simulink model "Intergration"  (R2018b)
settings: Solver=FixedStepDiscrete  StartTime=0.0  StopTime=inf  FixedStep=0.005  RelTol=1e-3
PostLoadFcn:
  | if any(exist('dsrtsu_mdlpostloadfcn', 'file') ~= 0), dsrtsu_mdlpostloadfcn('Execute', bdroot); end
values from neighbouring files (symbols this model uses):
  P_x165_On = 1.0    [CAN_Tx.sldd]
  P_x242_On = 1.0    [CAN_Tx.sldd]
  P_x246_On = 1.0    [CAN_Tx.sldd]
libraries: rtican x112, simulink x59
(part 29 of 31)

== system Intergration/Radar410_RX/Subsystem41/Subsystem29 ==
  In1 : Inport
  Bus Creator : BusCreator  Inputs=20  OutDataTypeStr=Bus: Obj_Data  NonVirtualBus=on
      settings: InheritFromInputs=off
  Bus Selector : BusSelector  OutputSignals=FRS_P1_27_Msg_CheckSum,FRS_P1_27_Msg_AliveCounter,FRS_P1_27_Obj_ExstProb,FRS_P1_27_Obj_XVelRel_Stdev,FRS_P1_27_Obj_XAccRel,FRS_P1_27_Obj_ObstacleProb,FRS_P1_27_Obj_MotionPattern,FRS_P1_27_Obj_YPos_Stdev,FRS_P1_27_Obj_ValidFlag,FRS_P1_27_Obj_XPos_Stdev,FRS_P1_27_Obj_UpdateFlag,FRS_P1_27_Obj_ID,FRS_P2_27_Msg_CheckSum,FRS_P2_27_Msg_AliveCounter,FRS_P2_27_Obj_MeasFlag,FRS_P2_27_Obj_YVelRel,FRS_P2_27_Obj_Type,FRS_P2_27_Obj_XPos,FRS_P2_27_Obj_YPos,FRS_P2_27_Obj_XVelRel
  Data Type Conversion{,1..19} (20 alike) : DataTypeConversion  OutDataTypeStr=single
  Out1 : Outport  OutDataTypeStr=Bus: Obj_Data
  wires:
  Data Type Conversion12/1 -> Bus Creator/13
  Bus Selector/5 -> Data Type Conversion4/1  "<FRS_P1_27_Obj_XAccRel>"
  Bus Selector/8 -> Data Type Conversion7/1  "<FRS_P1_27_Obj_YPos_Stdev>"
  Data Type Conversion15/1 -> Bus Creator/16
  Bus Selector/1 -> Data Type Conversion/1  "<FRS_P1_27_Msg_CheckSum>"
  Bus Selector/15 -> Data Type Conversion14/1  "<FRS_P2_27_Obj_MeasFlag>"
  Bus Selector/3 -> Data Type Conversion2/1  "<FRS_P1_27_Obj_ExstProb>"
  Bus Selector/13 -> Data Type Conversion12/1  "<FRS_P2_27_Msg_CheckSum>"
  Bus Selector/2 -> Data Type Conversion1/1  "<FRS_P1_27_Msg_AliveCounter>"
  Data Type Conversion11/1 -> Bus Creator/12
  Data Type Conversion5/1 -> Bus Creator/6
  Bus Selector/4 -> Data Type Conversion3/1  "<FRS_P1_27_Obj_XVelRel_Stdev>"
  Bus Selector/7 -> Data Type Conversion6/1  "<FRS_P1_27_Obj_MotionPattern>"
  Data Type Conversion9/1 -> Bus Creator/10
  Bus Selector/6 -> Data Type Conversion5/1  "<FRS_P1_27_Obj_ObstacleProb>"
  Data Type Conversion18/1 -> Bus Creator/19
  Bus Selector/11 -> Data Type Conversion10/1  "<FRS_P1_27_Obj_UpdateFlag>"
  Data Type Conversion17/1 -> Bus Creator/18
  Bus Selector/16 -> Data Type Conversion15/1  "<FRS_P2_27_Obj_YVelRel>"
  Data Type Conversion6/1 -> Bus Creator/7
  Bus Selector/12 -> Data Type Conversion11/1  "<FRS_P1_27_Obj_ID>"
  Data Type Conversion16/1 -> Bus Creator/17
  Bus Selector/9 -> Data Type Conversion8/1  "<FRS_P1_27_Obj_ValidFlag>"
  Bus Selector/17 -> Data Type Conversion16/1  "<FRS_P2_27_Obj_Type>"
  Bus Selector/10 -> Data Type Conversion9/1  "<FRS_P1_27_Obj_XPos_Stdev>"
  Data Type Conversion10/1 -> Bus Creator/11
  Bus Selector/14 -> Data Type Conversion13/1  "<FRS_P2_27_Msg_AliveCounter>"
  Bus Selector/19 -> Data Type Conversion18/1  "<FRS_P2_27_Obj_YPos>"
  Bus Selector/18 -> Data Type Conversion17/1  "<FRS_P2_27_Obj_XPos>"
  Bus Selector/20 -> Data Type Conversion19/1  "<FRS_P2_27_Obj_XVelRel>"
  In1/1 -> Bus Selector/1
  Bus Creator/1 -> Out1/1
  Data Type Conversion/1 -> Bus Creator/1
  Data Type Conversion2/1 -> Bus Creator/3
  Data Type Conversion13/1 -> Bus Creator/14
  Data Type Conversion1/1 -> Bus Creator/2
  Data Type Conversion4/1 -> Bus Creator/5
  Data Type Conversion3/1 -> Bus Creator/4
  Data Type Conversion7/1 -> Bus Creator/8
  Data Type Conversion8/1 -> Bus Creator/9
  Data Type Conversion14/1 -> Bus Creator/15
  Data Type Conversion19/1 -> Bus Creator/20

== system Intergration/Radar410_RX/Subsystem41/Subsystem3 ==
  In1 : Inport
  Bus Creator : BusCreator  Inputs=20  OutDataTypeStr=Bus: Obj_Data  NonVirtualBus=on
      settings: InheritFromInputs=off
  Bus Selector : BusSelector  OutputSignals=FRS_P1_03_Msg_CheckSum,FRS_P1_03_Msg_AliveCounter,FRS_P1_03_Obj_ExstProb,FRS_P1_03_Obj_XVelRel_Stdev,FRS_P1_03_Obj_XAccRel,FRS_P1_03_Obj_ObstacleProb,FRS_P1_03_Obj_MotionPattern,FRS_P1_03_Obj_YPos_Stdev,FRS_P1_03_Obj_ValidFlag,FRS_P1_03_Obj_XPos_Stdev,FRS_P1_03_Obj_UpdateFlag,FRS_P1_03_Obj_ID,FRS_P2_03_Msg_CheckSum,FRS_P2_03_Msg_AliveCounter,FRS_P2_03_Obj_MeasFlag,FRS_P2_03_Obj_YVelRel,FRS_P2_03_Obj_Type,FRS_P2_03_Obj_XPos,FRS_P2_03_Obj_YPos,FRS_P2_03_Obj_XVelRel
  Data Type Conversion{,1..19} (20 alike) : DataTypeConversion  OutDataTypeStr=single
  Out1 : Outport  OutDataTypeStr=Bus: Obj_Data
  wires:
  Data Type Conversion12/1 -> Bus Creator/13
  Bus Selector/5 -> Data Type Conversion4/1  "<FRS_P1_03_Obj_XAccRel>"
  Bus Selector/8 -> Data Type Conversion7/1  "<FRS_P1_03_Obj_YPos_Stdev>"
  Data Type Conversion15/1 -> Bus Creator/16
  Bus Selector/1 -> Data Type Conversion/1  "<FRS_P1_03_Msg_CheckSum>"
  Bus Selector/15 -> Data Type Conversion14/1  "<FRS_P2_03_Obj_MeasFlag>"
  Bus Selector/3 -> Data Type Conversion2/1  "<FRS_P1_03_Obj_ExstProb>"
  Bus Selector/13 -> Data Type Conversion12/1  "<FRS_P2_03_Msg_CheckSum>"
  Bus Selector/2 -> Data Type Conversion1/1  "<FRS_P1_03_Msg_AliveCounter>"
  Data Type Conversion11/1 -> Bus Creator/12
  Data Type Conversion5/1 -> Bus Creator/6
  Bus Selector/4 -> Data Type Conversion3/1  "<FRS_P1_03_Obj_XVelRel_Stdev>"
  Bus Selector/7 -> Data Type Conversion6/1  "<FRS_P1_03_Obj_MotionPattern>"
  Data Type Conversion9/1 -> Bus Creator/10
  Bus Selector/6 -> Data Type Conversion5/1  "<FRS_P1_03_Obj_ObstacleProb>"
  Data Type Conversion18/1 -> Bus Creator/19
  Bus Selector/11 -> Data Type Conversion10/1  "<FRS_P1_03_Obj_UpdateFlag>"
  Data Type Conversion17/1 -> Bus Creator/18
  Bus Selector/16 -> Data Type Conversion15/1  "<FRS_P2_03_Obj_YVelRel>"
  Data Type Conversion6/1 -> Bus Creator/7
  Bus Selector/12 -> Data Type Conversion11/1  "<FRS_P1_03_Obj_ID>"
  Data Type Conversion16/1 -> Bus Creator/17
  Bus Selector/9 -> Data Type Conversion8/1  "<FRS_P1_03_Obj_ValidFlag>"
  Bus Selector/17 -> Data Type Conversion16/1  "<FRS_P2_03_Obj_Type>"
  Bus Selector/10 -> Data Type Conversion9/1  "<FRS_P1_03_Obj_XPos_Stdev>"
  Data Type Conversion10/1 -> Bus Creator/11
  Bus Selector/14 -> Data Type Conversion13/1  "<FRS_P2_03_Msg_AliveCounter>"
  Bus Selector/19 -> Data Type Conversion18/1  "<FRS_P2_03_Obj_YPos>"
  Bus Selector/18 -> Data Type Conversion17/1  "<FRS_P2_03_Obj_XPos>"
  Bus Selector/20 -> Data Type Conversion19/1  "<FRS_P2_03_Obj_XVelRel>"
  In1/1 -> Bus Selector/1
  Bus Creator/1 -> Out1/1
  Data Type Conversion/1 -> Bus Creator/1
  Data Type Conversion2/1 -> Bus Creator/3
  Data Type Conversion13/1 -> Bus Creator/14
  Data Type Conversion1/1 -> Bus Creator/2
  Data Type Conversion4/1 -> Bus Creator/5
  Data Type Conversion3/1 -> Bus Creator/4
  Data Type Conversion7/1 -> Bus Creator/8
  Data Type Conversion8/1 -> Bus Creator/9
  Data Type Conversion14/1 -> Bus Creator/15
  Data Type Conversion19/1 -> Bus Creator/20

== system Intergration/Radar410_RX/Subsystem41/Subsystem30 ==
  In1 : Inport
  Bus Creator : BusCreator  Inputs=20  OutDataTypeStr=Bus: Obj_Data  NonVirtualBus=on
      settings: InheritFromInputs=off
  Bus Selector : BusSelector  OutputSignals=FRS_P1_28_Msg_CheckSum,FRS_P1_28_Msg_AliveCounter,FRS_P1_28_Obj_ExstProb,FRS_P1_28_Obj_XVelRel_Stdev,FRS_P1_28_Obj_XAccRel,FRS_P1_28_Obj_ObstacleProb,FRS_P1_28_Obj_MotionPattern,FRS_P1_28_Obj_YPos_Stdev,FRS_P1_28_Obj_ValidFlag,FRS_P1_28_Obj_XPos_Stdev,FRS_P1_28_Obj_UpdateFlag,FRS_P1_28_Obj_ID,FRS_P2_28_Msg_CheckSum,FRS_P2_28_Msg_AliveCounter,FRS_P2_28_Obj_MeasFlag,FRS_P2_28_Obj_YVelRel,FRS_P2_28_Obj_Type,FRS_P2_28_Obj_XPos,FRS_P2_28_Obj_YPos,FRS_P2_28_Obj_XVelRel
  Data Type Conversion{,1..19} (20 alike) : DataTypeConversion  OutDataTypeStr=single
  Out1 : Outport  OutDataTypeStr=Bus: Obj_Data
  wires:
  Data Type Conversion12/1 -> Bus Creator/13
  Bus Selector/5 -> Data Type Conversion4/1  "<FRS_P1_28_Obj_XAccRel>"
  Bus Selector/8 -> Data Type Conversion7/1  "<FRS_P1_28_Obj_YPos_Stdev>"
  Data Type Conversion15/1 -> Bus Creator/16
  Bus Selector/1 -> Data Type Conversion/1  "<FRS_P1_28_Msg_CheckSum>"
  Bus Selector/15 -> Data Type Conversion14/1  "<FRS_P2_28_Obj_MeasFlag>"
  Bus Selector/3 -> Data Type Conversion2/1  "<FRS_P1_28_Obj_ExstProb>"
  Bus Selector/13 -> Data Type Conversion12/1  "<FRS_P2_28_Msg_CheckSum>"
  Bus Selector/2 -> Data Type Conversion1/1  "<FRS_P1_28_Msg_AliveCounter>"
  Data Type Conversion11/1 -> Bus Creator/12
  Data Type Conversion5/1 -> Bus Creator/6
  Bus Selector/4 -> Data Type Conversion3/1  "<FRS_P1_28_Obj_XVelRel_Stdev>"
  Bus Selector/7 -> Data Type Conversion6/1  "<FRS_P1_28_Obj_MotionPattern>"
  Data Type Conversion9/1 -> Bus Creator/10
  Bus Selector/6 -> Data Type Conversion5/1  "<FRS_P1_28_Obj_ObstacleProb>"
  Data Type Conversion18/1 -> Bus Creator/19
  Bus Selector/11 -> Data Type Conversion10/1  "<FRS_P1_28_Obj_UpdateFlag>"
  Data Type Conversion17/1 -> Bus Creator/18
  Bus Selector/16 -> Data Type Conversion15/1  "<FRS_P2_28_Obj_YVelRel>"
  Data Type Conversion6/1 -> Bus Creator/7
  Bus Selector/12 -> Data Type Conversion11/1  "<FRS_P1_28_Obj_ID>"
  Data Type Conversion16/1 -> Bus Creator/17
  Bus Selector/9 -> Data Type Conversion8/1  "<FRS_P1_28_Obj_ValidFlag>"
  Bus Selector/17 -> Data Type Conversion16/1  "<FRS_P2_28_Obj_Type>"
  Bus Selector/10 -> Data Type Conversion9/1  "<FRS_P1_28_Obj_XPos_Stdev>"
  Data Type Conversion10/1 -> Bus Creator/11
  Bus Selector/14 -> Data Type Conversion13/1  "<FRS_P2_28_Msg_AliveCounter>"
  Bus Selector/19 -> Data Type Conversion18/1  "<FRS_P2_28_Obj_YPos>"
  Bus Selector/18 -> Data Type Conversion17/1  "<FRS_P2_28_Obj_XPos>"
  Bus Selector/20 -> Data Type Conversion19/1  "<FRS_P2_28_Obj_XVelRel>"
  In1/1 -> Bus Selector/1
  Bus Creator/1 -> Out1/1
  Data Type Conversion/1 -> Bus Creator/1
  Data Type Conversion2/1 -> Bus Creator/3
  Data Type Conversion13/1 -> Bus Creator/14
  Data Type Conversion1/1 -> Bus Creator/2
  Data Type Conversion4/1 -> Bus Creator/5
  Data Type Conversion3/1 -> Bus Creator/4
  Data Type Conversion7/1 -> Bus Creator/8
  Data Type Conversion8/1 -> Bus Creator/9
  Data Type Conversion14/1 -> Bus Creator/15
  Data Type Conversion19/1 -> Bus Creator/20

== system Intergration/Radar410_RX/Subsystem41/Subsystem31 ==
  In1 : Inport
  Bus Creator : BusCreator  Inputs=20  OutDataTypeStr=Bus: Obj_Data  NonVirtualBus=on
      settings: InheritFromInputs=off
  Bus Selector : BusSelector  OutputSignals=FRS_P1_29_Msg_CheckSum,FRS_P1_29_Msg_AliveCounter,FRS_P1_29_Obj_ExstProb,FRS_P1_29_Obj_XVelRel_Stdev,FRS_P1_29_Obj_XAccRel,FRS_P1_29_Obj_ObstacleProb,FRS_P1_29_Obj_MotionPattern,FRS_P1_29_Obj_YPos_Stdev,FRS_P1_29_Obj_ValidFlag,FRS_P1_29_Obj_XPos_Stdev,FRS_P1_29_Obj_UpdateFlag,FRS_P1_29_Obj_ID,FRS_P2_29_Msg_CheckSum,FRS_P2_29_Msg_AliveCounter,FRS_P2_29_Obj_MeasFlag,FRS_P2_29_Obj_YVelRel,FRS_P2_29_Obj_Type,FRS_P2_29_Obj_XPos,FRS_P2_29_Obj_YPos,FRS_P2_29_Obj_XVelRel
  Data Type Conversion{,1..19} (20 alike) : DataTypeConversion  OutDataTypeStr=single
  Out1 : Outport  OutDataTypeStr=Bus: Obj_Data
  wires:
  Data Type Conversion19/1 -> Bus Creator/20
  Data Type Conversion14/1 -> Bus Creator/15
  Data Type Conversion8/1 -> Bus Creator/9
  Data Type Conversion7/1 -> Bus Creator/8
  Data Type Conversion3/1 -> Bus Creator/4
  Data Type Conversion4/1 -> Bus Creator/5
  Data Type Conversion1/1 -> Bus Creator/2
  Data Type Conversion13/1 -> Bus Creator/14
  Data Type Conversion2/1 -> Bus Creator/3
  Data Type Conversion/1 -> Bus Creator/1
  Bus Creator/1 -> Out1/1
  In1/1 -> Bus Selector/1
  Bus Selector/20 -> Data Type Conversion19/1  "<FRS_P2_29_Obj_XVelRel>"
  Bus Selector/18 -> Data Type Conversion17/1  "<FRS_P2_29_Obj_XPos>"
  Bus Selector/19 -> Data Type Conversion18/1  "<FRS_P2_29_Obj_YPos>"
  Bus Selector/14 -> Data Type Conversion13/1  "<FRS_P2_29_Msg_AliveCounter>"
  Data Type Conversion10/1 -> Bus Creator/11
  Bus Selector/10 -> Data Type Conversion9/1  "<FRS_P1_29_Obj_XPos_Stdev>"
  Bus Selector/17 -> Data Type Conversion16/1  "<FRS_P2_29_Obj_Type>"
  Bus Selector/9 -> Data Type Conversion8/1  "<FRS_P1_29_Obj_ValidFlag>"
  Data Type Conversion16/1 -> Bus Creator/17
  Bus Selector/12 -> Data Type Conversion11/1  "<FRS_P1_29_Obj_ID>"
  Data Type Conversion6/1 -> Bus Creator/7
  Bus Selector/16 -> Data Type Conversion15/1  "<FRS_P2_29_Obj_YVelRel>"
  Data Type Conversion17/1 -> Bus Creator/18
  Bus Selector/11 -> Data Type Conversion10/1  "<FRS_P1_29_Obj_UpdateFlag>"
  Data Type Conversion18/1 -> Bus Creator/19
  Bus Selector/6 -> Data Type Conversion5/1  "<FRS_P1_29_Obj_ObstacleProb>"
  Data Type Conversion9/1 -> Bus Creator/10
  Bus Selector/7 -> Data Type Conversion6/1  "<FRS_P1_29_Obj_MotionPattern>"
  Bus Selector/4 -> Data Type Conversion3/1  "<FRS_P1_29_Obj_XVelRel_Stdev>"
  Data Type Conversion5/1 -> Bus Creator/6
  Data Type Conversion11/1 -> Bus Creator/12
  Bus Selector/2 -> Data Type Conversion1/1  "<FRS_P1_29_Msg_AliveCounter>"
  Bus Selector/13 -> Data Type Conversion12/1  "<FRS_P2_29_Msg_CheckSum>"
  Bus Selector/3 -> Data Type Conversion2/1  "<FRS_P1_29_Obj_ExstProb>"
  Bus Selector/15 -> Data Type Conversion14/1  "<FRS_P2_29_Obj_MeasFlag>"
  Bus Selector/1 -> Data Type Conversion/1  "<FRS_P1_29_Msg_CheckSum>"
  Data Type Conversion15/1 -> Bus Creator/16
  Bus Selector/8 -> Data Type Conversion7/1  "<FRS_P1_29_Obj_YPos_Stdev>"
  Bus Selector/5 -> Data Type Conversion4/1  "<FRS_P1_29_Obj_XAccRel>"
  Data Type Conversion12/1 -> Bus Creator/13

== system Intergration/Radar410_RX/Subsystem41/Subsystem32 ==
  In1 : Inport
  Bus Creator : BusCreator  Inputs=20  OutDataTypeStr=Bus: Obj_Data  NonVirtualBus=on
      settings: InheritFromInputs=off
  Bus Selector : BusSelector  OutputSignals=FRS_P1_30_Msg_CheckSum,FRS_P1_30_Msg_AliveCounter,FRS_P1_30_Obj_ExstProb,FRS_P1_30_Obj_XVelRel_Stdev,FRS_P1_30_Obj_XAccRel,FRS_P1_30_Obj_ObstacleProb,FRS_P1_30_Obj_MotionPattern,FRS_P1_30_Obj_YPos_Stdev,FRS_P1_30_Obj_ValidFlag,FRS_P1_30_Obj_XPos_Stdev,FRS_P1_30_Obj_UpdateFlag,FRS_P1_30_Obj_ID,FRS_P2_30_Msg_CheckSum,FRS_P2_30_Msg_AliveCounter,FRS_P2_30_Obj_MeasFlag,FRS_P2_30_Obj_YVelRel,FRS_P2_30_Obj_Type,FRS_P2_30_Obj_XPos,FRS_P2_30_Obj_YPos,FRS_P2_30_Obj_XVelRel
  Data Type Conversion{,1..19} (20 alike) : DataTypeConversion  OutDataTypeStr=single
  Out1 : Outport  OutDataTypeStr=Bus: Obj_Data
  wires:
  Data Type Conversion19/1 -> Bus Creator/20
  Data Type Conversion14/1 -> Bus Creator/15
  Data Type Conversion8/1 -> Bus Creator/9
  Data Type Conversion7/1 -> Bus Creator/8
  Data Type Conversion3/1 -> Bus Creator/4
  Data Type Conversion4/1 -> Bus Creator/5
  Data Type Conversion1/1 -> Bus Creator/2
  Data Type Conversion13/1 -> Bus Creator/14
  Data Type Conversion2/1 -> Bus Creator/3
  Data Type Conversion/1 -> Bus Creator/1
  Bus Creator/1 -> Out1/1
  In1/1 -> Bus Selector/1
  Bus Selector/20 -> Data Type Conversion19/1  "<FRS_P2_30_Obj_XVelRel>"
  Bus Selector/18 -> Data Type Conversion17/1  "<FRS_P2_30_Obj_XPos>"
  Bus Selector/19 -> Data Type Conversion18/1  "<FRS_P2_30_Obj_YPos>"
  Bus Selector/14 -> Data Type Conversion13/1  "<FRS_P2_30_Msg_AliveCounter>"
  Data Type Conversion10/1 -> Bus Creator/11
  Bus Selector/10 -> Data Type Conversion9/1  "<FRS_P1_30_Obj_XPos_Stdev>"
  Bus Selector/17 -> Data Type Conversion16/1  "<FRS_P2_30_Obj_Type>"
  Bus Selector/9 -> Data Type Conversion8/1  "<FRS_P1_30_Obj_ValidFlag>"
  Data Type Conversion16/1 -> Bus Creator/17
  Bus Selector/12 -> Data Type Conversion11/1  "<FRS_P1_30_Obj_ID>"
  Data Type Conversion6/1 -> Bus Creator/7
  Bus Selector/16 -> Data Type Conversion15/1  "<FRS_P2_30_Obj_YVelRel>"
  Data Type Conversion17/1 -> Bus Creator/18
  Bus Selector/11 -> Data Type Conversion10/1  "<FRS_P1_30_Obj_UpdateFlag>"
  Data Type Conversion18/1 -> Bus Creator/19
  Bus Selector/6 -> Data Type Conversion5/1  "<FRS_P1_30_Obj_ObstacleProb>"
  Data Type Conversion9/1 -> Bus Creator/10
  Bus Selector/7 -> Data Type Conversion6/1  "<FRS_P1_30_Obj_MotionPattern>"
  Bus Selector/4 -> Data Type Conversion3/1  "<FRS_P1_30_Obj_XVelRel_Stdev>"
  Data Type Conversion5/1 -> Bus Creator/6
  Data Type Conversion11/1 -> Bus Creator/12
  Bus Selector/2 -> Data Type Conversion1/1  "<FRS_P1_30_Msg_AliveCounter>"
  Bus Selector/13 -> Data Type Conversion12/1  "<FRS_P2_30_Msg_CheckSum>"
  Bus Selector/3 -> Data Type Conversion2/1  "<FRS_P1_30_Obj_ExstProb>"
  Bus Selector/15 -> Data Type Conversion14/1  "<FRS_P2_30_Obj_MeasFlag>"
  Bus Selector/1 -> Data Type Conversion/1  "<FRS_P1_30_Msg_CheckSum>"
  Data Type Conversion15/1 -> Bus Creator/16
  Bus Selector/8 -> Data Type Conversion7/1  "<FRS_P1_30_Obj_YPos_Stdev>"
  Bus Selector/5 -> Data Type Conversion4/1  "<FRS_P1_30_Obj_XAccRel>"
  Data Type Conversion12/1 -> Bus Creator/13

== system Intergration/Radar410_RX/Subsystem41/Subsystem33 ==
  In1 : Inport
  Bus Creator : BusCreator  Inputs=20  OutDataTypeStr=Bus: Obj_Data  NonVirtualBus=on
      settings: InheritFromInputs=off
  Bus Selector : BusSelector  OutputSignals=FRS_P1_31_Msg_CheckSum,FRS_P1_31_Msg_AliveCounter,FRS_P1_31_Obj_ExstProb,FRS_P1_31_Obj_XVelRel_Stdev,FRS_P1_31_Obj_XAccRel,FRS_P1_31_Obj_ObstacleProb,FRS_P1_31_Obj_MotionPattern,FRS_P1_31_Obj_YPos_Stdev,FRS_P1_31_Obj_ValidFlag,FRS_P1_31_Obj_XPos_Stdev,FRS_P1_31_Obj_UpdateFlag,FRS_P1_31_Obj_ID,FRS_P2_31_Msg_CheckSum,FRS_P2_31_Msg_AliveCounter,FRS_P2_31_Obj_MeasFlag,FRS_P2_31_Obj_YVelRel,FRS_P2_31_Obj_Type,FRS_P2_31_Obj_XPos,FRS_P2_31_Obj_YPos,FRS_P2_31_Obj_XVelRel
  Data Type Conversion{,1..19} (20 alike) : DataTypeConversion  OutDataTypeStr=single
  Out1 : Outport  OutDataTypeStr=Bus: Obj_Data
  wires:
  Data Type Conversion12/1 -> Bus Creator/13
  Bus Selector/5 -> Data Type Conversion4/1  "<FRS_P1_31_Obj_XAccRel>"
  Bus Selector/8 -> Data Type Conversion7/1  "<FRS_P1_31_Obj_YPos_Stdev>"
  Data Type Conversion15/1 -> Bus Creator/16
  Bus Selector/1 -> Data Type Conversion/1  "<FRS_P1_31_Msg_CheckSum>"
  Bus Selector/15 -> Data Type Conversion14/1  "<FRS_P2_31_Obj_MeasFlag>"
  Bus Selector/3 -> Data Type Conversion2/1  "<FRS_P1_31_Obj_ExstProb>"
  Bus Selector/13 -> Data Type Conversion12/1  "<FRS_P2_31_Msg_CheckSum>"
  Bus Selector/2 -> Data Type Conversion1/1  "<FRS_P1_31_Msg_AliveCounter>"
  Data Type Conversion11/1 -> Bus Creator/12
  Data Type Conversion5/1 -> Bus Creator/6
  Bus Selector/4 -> Data Type Conversion3/1  "<FRS_P1_31_Obj_XVelRel_Stdev>"
  Bus Selector/7 -> Data Type Conversion6/1  "<FRS_P1_31_Obj_MotionPattern>"
  Data Type Conversion9/1 -> Bus Creator/10
  Bus Selector/6 -> Data Type Conversion5/1  "<FRS_P1_31_Obj_ObstacleProb>"
  Data Type Conversion18/1 -> Bus Creator/19
  Bus Selector/11 -> Data Type Conversion10/1  "<FRS_P1_31_Obj_UpdateFlag>"
  Data Type Conversion17/1 -> Bus Creator/18
  Bus Selector/16 -> Data Type Conversion15/1  "<FRS_P2_31_Obj_YVelRel>"
  Data Type Conversion6/1 -> Bus Creator/7
  Bus Selector/12 -> Data Type Conversion11/1  "<FRS_P1_31_Obj_ID>"
  Data Type Conversion16/1 -> Bus Creator/17
  Bus Selector/9 -> Data Type Conversion8/1  "<FRS_P1_31_Obj_ValidFlag>"
  Bus Selector/17 -> Data Type Conversion16/1  "<FRS_P2_31_Obj_Type>"
  Bus Selector/10 -> Data Type Conversion9/1  "<FRS_P1_31_Obj_XPos_Stdev>"
  Data Type Conversion10/1 -> Bus Creator/11
  Bus Selector/14 -> Data Type Conversion13/1  "<FRS_P2_31_Msg_AliveCounter>"
  Bus Selector/19 -> Data Type Conversion18/1  "<FRS_P2_31_Obj_YPos>"
  Bus Selector/18 -> Data Type Conversion17/1  "<FRS_P2_31_Obj_XPos>"
  Bus Selector/20 -> Data Type Conversion19/1  "<FRS_P2_31_Obj_XVelRel>"
  In1/1 -> Bus Selector/1
  Bus Creator/1 -> Out1/1
  Data Type Conversion/1 -> Bus Creator/1
  Data Type Conversion2/1 -> Bus Creator/3
  Data Type Conversion13/1 -> Bus Creator/14
  Data Type Conversion1/1 -> Bus Creator/2
  Data Type Conversion4/1 -> Bus Creator/5
  Data Type Conversion3/1 -> Bus Creator/4
  Data Type Conversion7/1 -> Bus Creator/8
  Data Type Conversion8/1 -> Bus Creator/9
  Data Type Conversion14/1 -> Bus Creator/15
  Data Type Conversion19/1 -> Bus Creator/20

== system Intergration/Radar410_RX/Subsystem41/Subsystem34 ==
  In1 : Inport
  Bus Creator : BusCreator  Inputs=20  OutDataTypeStr=Bus: Obj_Data  NonVirtualBus=on
      settings: InheritFromInputs=off
  Bus Selector : BusSelector  OutputSignals=FRS_P1_32_Msg_CheckSum,FRS_P1_32_Msg_AliveCounter,FRS_P1_32_Obj_ExstProb,FRS_P1_32_Obj_XVelRel_Stdev,FRS_P1_32_Obj_XAccRel,FRS_P1_32_Obj_ObstacleProb,FRS_P1_32_Obj_MotionPattern,FRS_P1_32_Obj_YPos_Stdev,FRS_P1_32_Obj_ValidFlag,FRS_P1_32_Obj_XPos_Stdev,FRS_P1_32_Obj_UpdateFlag,FRS_P1_32_Obj_ID,FRS_P2_32_Msg_CheckSum,FRS_P2_32_Msg_AliveCounter,FRS_P2_32_Obj_MeasFlag,FRS_P2_32_Obj_YVelRel,FRS_P2_32_Obj_Type,FRS_P2_32_Obj_XPos,FRS_P2_32_Obj_YPos,FRS_P2_32_Obj_XVelRel
  Data Type Conversion{,1..19} (20 alike) : DataTypeConversion  OutDataTypeStr=single
  Out1 : Outport  OutDataTypeStr=Bus: Obj_Data
  wires:
  Data Type Conversion12/1 -> Bus Creator/13
  Bus Selector/5 -> Data Type Conversion4/1  "<FRS_P1_32_Obj_XAccRel>"
  Bus Selector/8 -> Data Type Conversion7/1  "<FRS_P1_32_Obj_YPos_Stdev>"
  Data Type Conversion15/1 -> Bus Creator/16
  Bus Selector/1 -> Data Type Conversion/1  "<FRS_P1_32_Msg_CheckSum>"
  Bus Selector/15 -> Data Type Conversion14/1  "<FRS_P2_32_Obj_MeasFlag>"
  Bus Selector/3 -> Data Type Conversion2/1  "<FRS_P1_32_Obj_ExstProb>"
  Bus Selector/13 -> Data Type Conversion12/1  "<FRS_P2_32_Msg_CheckSum>"
  Bus Selector/2 -> Data Type Conversion1/1  "<FRS_P1_32_Msg_AliveCounter>"
  Data Type Conversion11/1 -> Bus Creator/12
  Data Type Conversion5/1 -> Bus Creator/6
  Bus Selector/4 -> Data Type Conversion3/1  "<FRS_P1_32_Obj_XVelRel_Stdev>"
  Bus Selector/7 -> Data Type Conversion6/1  "<FRS_P1_32_Obj_MotionPattern>"
  Data Type Conversion9/1 -> Bus Creator/10
  Bus Selector/6 -> Data Type Conversion5/1  "<FRS_P1_32_Obj_ObstacleProb>"
  Data Type Conversion18/1 -> Bus Creator/19
  Bus Selector/11 -> Data Type Conversion10/1  "<FRS_P1_32_Obj_UpdateFlag>"
  Data Type Conversion17/1 -> Bus Creator/18
  Bus Selector/16 -> Data Type Conversion15/1  "<FRS_P2_32_Obj_YVelRel>"
  Data Type Conversion6/1 -> Bus Creator/7
  Bus Selector/12 -> Data Type Conversion11/1  "<FRS_P1_32_Obj_ID>"
  Data Type Conversion16/1 -> Bus Creator/17
  Bus Selector/9 -> Data Type Conversion8/1  "<FRS_P1_32_Obj_ValidFlag>"
  Bus Selector/17 -> Data Type Conversion16/1  "<FRS_P2_32_Obj_Type>"
  Bus Selector/10 -> Data Type Conversion9/1  "<FRS_P1_32_Obj_XPos_Stdev>"
  Data Type Conversion10/1 -> Bus Creator/11
  Bus Selector/14 -> Data Type Conversion13/1  "<FRS_P2_32_Msg_AliveCounter>"
  Bus Selector/19 -> Data Type Conversion18/1  "<FRS_P2_32_Obj_YPos>"
  Bus Selector/18 -> Data Type Conversion17/1  "<FRS_P2_32_Obj_XPos>"
  Bus Selector/20 -> Data Type Conversion19/1  "<FRS_P2_32_Obj_XVelRel>"
  In1/1 -> Bus Selector/1
  Bus Creator/1 -> Out1/1
  Data Type Conversion/1 -> Bus Creator/1
  Data Type Conversion2/1 -> Bus Creator/3
  Data Type Conversion13/1 -> Bus Creator/14
  Data Type Conversion1/1 -> Bus Creator/2
  Data Type Conversion4/1 -> Bus Creator/5
  Data Type Conversion3/1 -> Bus Creator/4
  Data Type Conversion7/1 -> Bus Creator/8
  Data Type Conversion8/1 -> Bus Creator/9
  Data Type Conversion14/1 -> Bus Creator/15
  Data Type Conversion19/1 -> Bus Creator/20

== system Intergration/Radar410_RX/Subsystem41/Subsystem35 ==
  In1 : Inport
  Bus Creator : BusCreator  Inputs=20  OutDataTypeStr=Bus: Obj_Data  NonVirtualBus=on
      settings: InheritFromInputs=off
  Bus Selector : BusSelector  OutputSignals=FRS_P1_33_Msg_CheckSum,FRS_P1_33_Msg_AliveCounter,FRS_P1_33_Obj_ExstProb,FRS_P1_33_Obj_XVelRel_Stdev,FRS_P1_33_Obj_XAccRel,FRS_P1_33_Obj_ObstacleProb,FRS_P1_33_Obj_MotionPattern,FRS_P1_33_Obj_YPos_Stdev,FRS_P1_33_Obj_ValidFlag,FRS_P1_33_Obj_XPos_Stdev,FRS_P1_33_Obj_UpdateFlag,FRS_P1_33_Obj_ID,FRS_P2_33_Msg_CheckSum,FRS_P2_33_Msg_AliveCounter,FRS_P2_33_Obj_MeasFlag,FRS_P2_33_Obj_YVelRel,FRS_P2_33_Obj_Type,FRS_P2_33_Obj_XPos,FRS_P2_33_Obj_YPos,FRS_P2_33_Obj_XVelRel
  Data Type Conversion{,1..19} (20 alike) : DataTypeConversion  OutDataTypeStr=single
  Out1 : Outport  OutDataTypeStr=Bus: Obj_Data
  wires:
  Data Type Conversion19/1 -> Bus Creator/20
  Data Type Conversion14/1 -> Bus Creator/15
  Data Type Conversion8/1 -> Bus Creator/9
  Data Type Conversion7/1 -> Bus Creator/8
  Data Type Conversion3/1 -> Bus Creator/4
  Data Type Conversion4/1 -> Bus Creator/5
  Data Type Conversion1/1 -> Bus Creator/2
  Data Type Conversion13/1 -> Bus Creator/14
  Data Type Conversion2/1 -> Bus Creator/3
  Data Type Conversion/1 -> Bus Creator/1
  Bus Creator/1 -> Out1/1
  In1/1 -> Bus Selector/1
  Bus Selector/20 -> Data Type Conversion19/1  "<FRS_P2_33_Obj_XVelRel>"
  Bus Selector/18 -> Data Type Conversion17/1  "<FRS_P2_33_Obj_XPos>"
  Bus Selector/19 -> Data Type Conversion18/1  "<FRS_P2_33_Obj_YPos>"
  Bus Selector/14 -> Data Type Conversion13/1  "<FRS_P2_33_Msg_AliveCounter>"
  Data Type Conversion10/1 -> Bus Creator/11
  Bus Selector/10 -> Data Type Conversion9/1  "<FRS_P1_33_Obj_XPos_Stdev>"
  Bus Selector/17 -> Data Type Conversion16/1  "<FRS_P2_33_Obj_Type>"
  Bus Selector/9 -> Data Type Conversion8/1  "<FRS_P1_33_Obj_ValidFlag>"
  Data Type Conversion16/1 -> Bus Creator/17
  Bus Selector/12 -> Data Type Conversion11/1  "<FRS_P1_33_Obj_ID>"
  Data Type Conversion6/1 -> Bus Creator/7
  Bus Selector/16 -> Data Type Conversion15/1  "<FRS_P2_33_Obj_YVelRel>"
  Data Type Conversion17/1 -> Bus Creator/18
  Bus Selector/11 -> Data Type Conversion10/1  "<FRS_P1_33_Obj_UpdateFlag>"
  Data Type Conversion18/1 -> Bus Creator/19
  Bus Selector/6 -> Data Type Conversion5/1  "<FRS_P1_33_Obj_ObstacleProb>"
  Data Type Conversion9/1 -> Bus Creator/10
  Bus Selector/7 -> Data Type Conversion6/1  "<FRS_P1_33_Obj_MotionPattern>"
  Bus Selector/4 -> Data Type Conversion3/1  "<FRS_P1_33_Obj_XVelRel_Stdev>"
  Data Type Conversion5/1 -> Bus Creator/6
  Data Type Conversion11/1 -> Bus Creator/12
  Bus Selector/2 -> Data Type Conversion1/1  "<FRS_P1_33_Msg_AliveCounter>"
  Bus Selector/13 -> Data Type Conversion12/1  "<FRS_P2_33_Msg_CheckSum>"
  Bus Selector/3 -> Data Type Conversion2/1  "<FRS_P1_33_Obj_ExstProb>"
  Bus Selector/15 -> Data Type Conversion14/1  "<FRS_P2_33_Obj_MeasFlag>"
  Bus Selector/1 -> Data Type Conversion/1  "<FRS_P1_33_Msg_CheckSum>"
  Data Type Conversion15/1 -> Bus Creator/16
  Bus Selector/8 -> Data Type Conversion7/1  "<FRS_P1_33_Obj_YPos_Stdev>"
  Bus Selector/5 -> Data Type Conversion4/1  "<FRS_P1_33_Obj_XAccRel>"
  Data Type Conversion12/1 -> Bus Creator/13

== system Intergration/Radar410_RX/Subsystem41/Subsystem36 ==
  In1 : Inport
  Bus Creator : BusCreator  Inputs=20  OutDataTypeStr=Bus: Obj_Data  NonVirtualBus=on
      settings: InheritFromInputs=off
  Bus Selector : BusSelector  OutputSignals=FRS_P1_38_Msg_CheckSum,FRS_P1_38_Msg_AliveCounter,FRS_P1_38_Obj_ExstProb,FRS_P1_38_Obj_XVelRel_Stdev,FRS_P1_38_Obj_XAccRel,FRS_P1_38_Obj_ObstacleProb,FRS_P1_38_Obj_MotionPattern,FRS_P1_38_Obj_YPos_Stdev,FRS_P1_38_Obj_ValidFlag,FRS_P1_38_Obj_XPos_Stdev,FRS_P1_38_Obj_UpdateFlag,FRS_P1_38_Obj_ID,FRS_P2_38_Msg_CheckSum,FRS_P2_38_Msg_AliveCounter,FRS_P2_38_Obj_MeasFlag,FRS_P2_38_Obj_YVelRel,FRS_P2_38_Obj_Type,FRS_P2_38_Obj_XPos,FRS_P2_38_Obj_YPos,FRS_P2_38_Obj_XVelRel
  Data Type Conversion{,1..19} (20 alike) : DataTypeConversion  OutDataTypeStr=single
  Out1 : Outport  OutDataTypeStr=Bus: Obj_Data
  wires:
  Data Type Conversion12/1 -> Bus Creator/13
  Bus Selector/5 -> Data Type Conversion4/1  "<FRS_P1_38_Obj_XAccRel>"
  Bus Selector/8 -> Data Type Conversion7/1  "<FRS_P1_38_Obj_YPos_Stdev>"
  Data Type Conversion15/1 -> Bus Creator/16
  Bus Selector/1 -> Data Type Conversion/1  "<FRS_P1_38_Msg_CheckSum>"
  Bus Selector/15 -> Data Type Conversion14/1  "<FRS_P2_38_Obj_MeasFlag>"
  Bus Selector/3 -> Data Type Conversion2/1  "<FRS_P1_38_Obj_ExstProb>"
  Bus Selector/13 -> Data Type Conversion12/1  "<FRS_P2_38_Msg_CheckSum>"
  Bus Selector/2 -> Data Type Conversion1/1  "<FRS_P1_38_Msg_AliveCounter>"
  Data Type Conversion11/1 -> Bus Creator/12
  Data Type Conversion5/1 -> Bus Creator/6
  Bus Selector/4 -> Data Type Conversion3/1  "<FRS_P1_38_Obj_XVelRel_Stdev>"
  Bus Selector/7 -> Data Type Conversion6/1  "<FRS_P1_38_Obj_MotionPattern>"
  Data Type Conversion9/1 -> Bus Creator/10
  Bus Selector/6 -> Data Type Conversion5/1  "<FRS_P1_38_Obj_ObstacleProb>"
  Data Type Conversion18/1 -> Bus Creator/19
  Bus Selector/11 -> Data Type Conversion10/1  "<FRS_P1_38_Obj_UpdateFlag>"
  Data Type Conversion17/1 -> Bus Creator/18
  Bus Selector/16 -> Data Type Conversion15/1  "<FRS_P2_38_Obj_YVelRel>"
  Data Type Conversion6/1 -> Bus Creator/7
  Bus Selector/12 -> Data Type Conversion11/1  "<FRS_P1_38_Obj_ID>"
  Data Type Conversion16/1 -> Bus Creator/17
  Bus Selector/9 -> Data Type Conversion8/1  "<FRS_P1_38_Obj_ValidFlag>"
  Bus Selector/17 -> Data Type Conversion16/1  "<FRS_P2_38_Obj_Type>"
  Bus Selector/10 -> Data Type Conversion9/1  "<FRS_P1_38_Obj_XPos_Stdev>"
  Data Type Conversion10/1 -> Bus Creator/11
  Bus Selector/14 -> Data Type Conversion13/1  "<FRS_P2_38_Msg_AliveCounter>"
  Bus Selector/19 -> Data Type Conversion18/1  "<FRS_P2_38_Obj_YPos>"
  Bus Selector/18 -> Data Type Conversion17/1  "<FRS_P2_38_Obj_XPos>"
  Bus Selector/20 -> Data Type Conversion19/1  "<FRS_P2_38_Obj_XVelRel>"
  In1/1 -> Bus Selector/1
  Bus Creator/1 -> Out1/1
  Data Type Conversion/1 -> Bus Creator/1
  Data Type Conversion2/1 -> Bus Creator/3
  Data Type Conversion13/1 -> Bus Creator/14
  Data Type Conversion1/1 -> Bus Creator/2
  Data Type Conversion4/1 -> Bus Creator/5
  Data Type Conversion3/1 -> Bus Creator/4
  Data Type Conversion7/1 -> Bus Creator/8
  Data Type Conversion8/1 -> Bus Creator/9
  Data Type Conversion14/1 -> Bus Creator/15
  Data Type Conversion19/1 -> Bus Creator/20

== system Intergration/Radar410_RX/Subsystem41/Subsystem37 ==
  In1 : Inport
  Bus Creator : BusCreator  Inputs=20  OutDataTypeStr=Bus: Obj_Data  NonVirtualBus=on
      settings: InheritFromInputs=off
  Bus Selector : BusSelector  OutputSignals=FRS_P1_39_Msg_CheckSum,FRS_P1_39_Msg_AliveCounter,FRS_P1_39_Obj_ExstProb,FRS_P1_39_Obj_XVelRel_Stdev,FRS_P1_39_Obj_XAccRel,FRS_P1_39_Obj_ObstacleProb,FRS_P1_39_Obj_MotionPattern,FRS_P1_39_Obj_YPos_Stdev,FRS_P1_39_Obj_ValidFlag,FRS_P1_39_Obj_XPos_Stdev,FRS_P1_39_Obj_UpdateFlag,FRS_P1_39_Obj_ID,FRS_P2_39_Msg_CheckSum,FRS_P2_39_Msg_AliveCounter,FRS_P2_39_Obj_MeasFlag,FRS_P2_39_Obj_YVelRel,FRS_P2_39_Obj_Type,FRS_P2_39_Obj_XPos,FRS_P2_39_Obj_YPos,FRS_P2_39_Obj_XVelRel
  Data Type Conversion{,1..19} (20 alike) : DataTypeConversion  OutDataTypeStr=single
  Out1 : Outport  OutDataTypeStr=Bus: Obj_Data
  wires:
  Data Type Conversion19/1 -> Bus Creator/20
  Data Type Conversion14/1 -> Bus Creator/15
  Data Type Conversion8/1 -> Bus Creator/9
  Data Type Conversion7/1 -> Bus Creator/8
  Data Type Conversion3/1 -> Bus Creator/4
  Data Type Conversion4/1 -> Bus Creator/5
  Data Type Conversion1/1 -> Bus Creator/2
  Data Type Conversion13/1 -> Bus Creator/14
  Data Type Conversion2/1 -> Bus Creator/3
  Data Type Conversion/1 -> Bus Creator/1
  Bus Creator/1 -> Out1/1
  In1/1 -> Bus Selector/1
  Bus Selector/20 -> Data Type Conversion19/1  "<FRS_P2_39_Obj_XVelRel>"
  Bus Selector/18 -> Data Type Conversion17/1  "<FRS_P2_39_Obj_XPos>"
  Bus Selector/19 -> Data Type Conversion18/1  "<FRS_P2_39_Obj_YPos>"
  Bus Selector/14 -> Data Type Conversion13/1  "<FRS_P2_39_Msg_AliveCounter>"
  Data Type Conversion10/1 -> Bus Creator/11
  Bus Selector/10 -> Data Type Conversion9/1  "<FRS_P1_39_Obj_XPos_Stdev>"
  Bus Selector/17 -> Data Type Conversion16/1  "<FRS_P2_39_Obj_Type>"
  Bus Selector/9 -> Data Type Conversion8/1  "<FRS_P1_39_Obj_ValidFlag>"
  Data Type Conversion16/1 -> Bus Creator/17
  Bus Selector/12 -> Data Type Conversion11/1  "<FRS_P1_39_Obj_ID>"
  Data Type Conversion6/1 -> Bus Creator/7
  Bus Selector/16 -> Data Type Conversion15/1  "<FRS_P2_39_Obj_YVelRel>"
  Data Type Conversion17/1 -> Bus Creator/18
  Bus Selector/11 -> Data Type Conversion10/1  "<FRS_P1_39_Obj_UpdateFlag>"
  Data Type Conversion18/1 -> Bus Creator/19
  Bus Selector/6 -> Data Type Conversion5/1  "<FRS_P1_39_Obj_ObstacleProb>"
  Data Type Conversion9/1 -> Bus Creator/10
  Bus Selector/7 -> Data Type Conversion6/1  "<FRS_P1_39_Obj_MotionPattern>"
  Bus Selector/4 -> Data Type Conversion3/1  "<FRS_P1_39_Obj_XVelRel_Stdev>"
  Data Type Conversion5/1 -> Bus Creator/6
  Data Type Conversion11/1 -> Bus Creator/12
  Bus Selector/2 -> Data Type Conversion1/1  "<FRS_P1_39_Msg_AliveCounter>"
  Bus Selector/13 -> Data Type Conversion12/1  "<FRS_P2_39_Msg_CheckSum>"
  Bus Selector/3 -> Data Type Conversion2/1  "<FRS_P1_39_Obj_ExstProb>"
  Bus Selector/15 -> Data Type Conversion14/1  "<FRS_P2_39_Obj_MeasFlag>"
  Bus Selector/1 -> Data Type Conversion/1  "<FRS_P1_39_Msg_CheckSum>"
  Data Type Conversion15/1 -> Bus Creator/16
  Bus Selector/8 -> Data Type Conversion7/1  "<FRS_P1_39_Obj_YPos_Stdev>"
  Bus Selector/5 -> Data Type Conversion4/1  "<FRS_P1_39_Obj_XAccRel>"
  Data Type Conversion12/1 -> Bus Creator/13

== system Intergration/Radar410_RX/Subsystem41/Subsystem38 ==
  In1 : Inport
  Bus Creator : BusCreator  Inputs=20  OutDataTypeStr=Bus: Obj_Data  NonVirtualBus=on
      settings: InheritFromInputs=off
  Bus Selector : BusSelector  OutputSignals=FRS_P1_36_Msg_CheckSum,FRS_P1_36_Msg_AliveCounter,FRS_P1_36_Obj_ExstProb,FRS_P1_36_Obj_XVelRel_Stdev,FRS_P1_36_Obj_XAccRel,FRS_P1_36_Obj_ObstacleProb,FRS_P1_36_Obj_MotionPattern,FRS_P1_36_Obj_YPos_Stdev,FRS_P1_36_Obj_ValidFlag,FRS_P1_36_Obj_XPos_Stdev,FRS_P1_36_Obj_UpdateFlag,FRS_P1_36_Obj_ID,FRS_P2_36_Msg_CheckSum,FRS_P2_36_Msg_AliveCounter,FRS_P2_36_Obj_MeasFlag,FRS_P2_36_Obj_YVelRel,FRS_P2_36_Obj_Type,FRS_P2_36_Obj_XPos,FRS_P2_36_Obj_YPos,FRS_P2_36_Obj_XVelRel
  Data Type Conversion{,1..19} (20 alike) : DataTypeConversion  OutDataTypeStr=single
  Out1 : Outport  OutDataTypeStr=Bus: Obj_Data
  wires:
  Data Type Conversion19/1 -> Bus Creator/20
  Data Type Conversion14/1 -> Bus Creator/15
  Data Type Conversion8/1 -> Bus Creator/9
  Data Type Conversion7/1 -> Bus Creator/8
  Data Type Conversion3/1 -> Bus Creator/4
  Data Type Conversion4/1 -> Bus Creator/5
  Data Type Conversion1/1 -> Bus Creator/2
  Data Type Conversion13/1 -> Bus Creator/14
  Data Type Conversion2/1 -> Bus Creator/3
  Data Type Conversion/1 -> Bus Creator/1
  Bus Creator/1 -> Out1/1
  In1/1 -> Bus Selector/1
  Bus Selector/20 -> Data Type Conversion19/1  "<FRS_P2_36_Obj_XVelRel>"
  Bus Selector/18 -> Data Type Conversion17/1  "<FRS_P2_36_Obj_XPos>"
  Bus Selector/19 -> Data Type Conversion18/1  "<FRS_P2_36_Obj_YPos>"
  Bus Selector/14 -> Data Type Conversion13/1  "<FRS_P2_36_Msg_AliveCounter>"
  Data Type Conversion10/1 -> Bus Creator/11
  Bus Selector/10 -> Data Type Conversion9/1  "<FRS_P1_36_Obj_XPos_Stdev>"
  Bus Selector/17 -> Data Type Conversion16/1  "<FRS_P2_36_Obj_Type>"
  Bus Selector/9 -> Data Type Conversion8/1  "<FRS_P1_36_Obj_ValidFlag>"
  Data Type Conversion16/1 -> Bus Creator/17
  Bus Selector/12 -> Data Type Conversion11/1  "<FRS_P1_36_Obj_ID>"
  Data Type Conversion6/1 -> Bus Creator/7
  Bus Selector/16 -> Data Type Conversion15/1  "<FRS_P2_36_Obj_YVelRel>"
  Data Type Conversion17/1 -> Bus Creator/18
  Bus Selector/11 -> Data Type Conversion10/1  "<FRS_P1_36_Obj_UpdateFlag>"
  Data Type Conversion18/1 -> Bus Creator/19
  Bus Selector/6 -> Data Type Conversion5/1  "<FRS_P1_36_Obj_ObstacleProb>"
  Data Type Conversion9/1 -> Bus Creator/10
  Bus Selector/7 -> Data Type Conversion6/1  "<FRS_P1_36_Obj_MotionPattern>"
  Bus Selector/4 -> Data Type Conversion3/1  "<FRS_P1_36_Obj_XVelRel_Stdev>"
  Data Type Conversion5/1 -> Bus Creator/6
  Data Type Conversion11/1 -> Bus Creator/12
  Bus Selector/2 -> Data Type Conversion1/1  "<FRS_P1_36_Msg_AliveCounter>"
  Bus Selector/13 -> Data Type Conversion12/1  "<FRS_P2_36_Msg_CheckSum>"
  Bus Selector/3 -> Data Type Conversion2/1  "<FRS_P1_36_Obj_ExstProb>"
  Bus Selector/15 -> Data Type Conversion14/1  "<FRS_P2_36_Obj_MeasFlag>"
  Bus Selector/1 -> Data Type Conversion/1  "<FRS_P1_36_Msg_CheckSum>"
  Data Type Conversion15/1 -> Bus Creator/16
  Bus Selector/8 -> Data Type Conversion7/1  "<FRS_P1_36_Obj_YPos_Stdev>"
  Bus Selector/5 -> Data Type Conversion4/1  "<FRS_P1_36_Obj_XAccRel>"
  Data Type Conversion12/1 -> Bus Creator/13

== system Intergration/Radar410_RX/Subsystem41/Subsystem39 ==
  In1 : Inport
  Bus Creator : BusCreator  Inputs=20  OutDataTypeStr=Bus: Obj_Data  NonVirtualBus=on
      settings: InheritFromInputs=off
  Bus Selector : BusSelector  OutputSignals=FRS_P1_37_Msg_CheckSum,FRS_P1_37_Msg_AliveCounter,FRS_P1_37_Obj_ExstProb,FRS_P1_37_Obj_XVelRel_Stdev,FRS_P1_37_Obj_XAccRel,FRS_P1_37_Obj_ObstacleProb,FRS_P1_37_Obj_MotionPattern,FRS_P1_37_Obj_YPos_Stdev,FRS_P1_37_Obj_ValidFlag,FRS_P1_37_Obj_XPos_Stdev,FRS_P1_37_Obj_UpdateFlag,FRS_P1_37_Obj_ID,FRS_P2_37_Msg_CheckSum,FRS_P2_37_Msg_AliveCounter,FRS_P2_37_Obj_MeasFlag,FRS_P2_37_Obj_YVelRel,FRS_P2_37_Obj_Type,FRS_P2_37_Obj_XPos,FRS_P2_37_Obj_YPos,FRS_P2_37_Obj_XVelRel
  Data Type Conversion{,1..19} (20 alike) : DataTypeConversion  OutDataTypeStr=single
  Out1 : Outport  OutDataTypeStr=Bus: Obj_Data
  wires:
  Data Type Conversion12/1 -> Bus Creator/13
  Bus Selector/5 -> Data Type Conversion4/1  "<FRS_P1_37_Obj_XAccRel>"
  Bus Selector/8 -> Data Type Conversion7/1  "<FRS_P1_37_Obj_YPos_Stdev>"
  Data Type Conversion15/1 -> Bus Creator/16
  Bus Selector/1 -> Data Type Conversion/1  "<FRS_P1_37_Msg_CheckSum>"
  Bus Selector/15 -> Data Type Conversion14/1  "<FRS_P2_37_Obj_MeasFlag>"
  Bus Selector/3 -> Data Type Conversion2/1  "<FRS_P1_37_Obj_ExstProb>"
  Bus Selector/13 -> Data Type Conversion12/1  "<FRS_P2_37_Msg_CheckSum>"
  Bus Selector/2 -> Data Type Conversion1/1  "<FRS_P1_37_Msg_AliveCounter>"
  Data Type Conversion11/1 -> Bus Creator/12
  Data Type Conversion5/1 -> Bus Creator/6
  Bus Selector/4 -> Data Type Conversion3/1  "<FRS_P1_37_Obj_XVelRel_Stdev>"
  Bus Selector/7 -> Data Type Conversion6/1  "<FRS_P1_37_Obj_MotionPattern>"
  Data Type Conversion9/1 -> Bus Creator/10
  Bus Selector/6 -> Data Type Conversion5/1  "<FRS_P1_37_Obj_ObstacleProb>"
  Data Type Conversion18/1 -> Bus Creator/19
  Bus Selector/11 -> Data Type Conversion10/1  "<FRS_P1_37_Obj_UpdateFlag>"
  Data Type Conversion17/1 -> Bus Creator/18
  Bus Selector/16 -> Data Type Conversion15/1  "<FRS_P2_37_Obj_YVelRel>"
  Data Type Conversion6/1 -> Bus Creator/7
  Bus Selector/12 -> Data Type Conversion11/1  "<FRS_P1_37_Obj_ID>"
  Data Type Conversion16/1 -> Bus Creator/17
  Bus Selector/9 -> Data Type Conversion8/1  "<FRS_P1_37_Obj_ValidFlag>"
  Bus Selector/17 -> Data Type Conversion16/1  "<FRS_P2_37_Obj_Type>"
  Bus Selector/10 -> Data Type Conversion9/1  "<FRS_P1_37_Obj_XPos_Stdev>"
  Data Type Conversion10/1 -> Bus Creator/11
  Bus Selector/14 -> Data Type Conversion13/1  "<FRS_P2_37_Msg_AliveCounter>"
  Bus Selector/19 -> Data Type Conversion18/1  "<FRS_P2_37_Obj_YPos>"
  Bus Selector/18 -> Data Type Conversion17/1  "<FRS_P2_37_Obj_XPos>"
  Bus Selector/20 -> Data Type Conversion19/1  "<FRS_P2_37_Obj_XVelRel>"
  In1/1 -> Bus Selector/1
  Bus Creator/1 -> Out1/1
  Data Type Conversion/1 -> Bus Creator/1
  Data Type Conversion2/1 -> Bus Creator/3
  Data Type Conversion13/1 -> Bus Creator/14
  Data Type Conversion1/1 -> Bus Creator/2
  Data Type Conversion4/1 -> Bus Creator/5
  Data Type Conversion3/1 -> Bus Creator/4
  Data Type Conversion7/1 -> Bus Creator/8
  Data Type Conversion8/1 -> Bus Creator/9
  Data Type Conversion14/1 -> Bus Creator/15
  Data Type Conversion19/1 -> Bus Creator/20

== system Intergration/Radar410_RX/Subsystem41/Subsystem4 ==
  In1 : Inport
  Bus Creator : BusCreator  Inputs=20  OutDataTypeStr=Bus: Obj_Data  NonVirtualBus=on
      settings: InheritFromInputs=off
  Bus Selector : BusSelector  OutputSignals=FRS_P1_04_Msg_CheckSum,FRS_P1_04_Msg_AliveCounter,FRS_P1_04_Obj_ExstProb,FRS_P1_04_Obj_XVelRel_Stdev,FRS_P1_04_Obj_XAccRel,FRS_P1_04_Obj_ObstacleProb,FRS_P1_04_Obj_MotionPattern,FRS_P1_04_Obj_YPos_Stdev,FRS_P1_04_Obj_ValidFlag,FRS_P1_04_Obj_XPos_Stdev,FRS_P1_04_Obj_UpdateFlag,FRS_P1_04_Obj_ID,FRS_P2_04_Msg_CheckSum,FRS_P2_04_Msg_AliveCounter,FRS_P2_04_Obj_MeasFlag,FRS_P2_04_Obj_YVelRel,FRS_P2_04_Obj_Type,FRS_P2_04_Obj_XPos,FRS_P2_04_Obj_YPos,FRS_P2_04_Obj_XVelRel
  Data Type Conversion{,1..19} (20 alike) : DataTypeConversion  OutDataTypeStr=single
  Out1 : Outport  OutDataTypeStr=Bus: Obj_Data
  wires:
  Data Type Conversion12/1 -> Bus Creator/13
  Bus Selector/5 -> Data Type Conversion4/1  "<FRS_P1_04_Obj_XAccRel>"
  Bus Selector/8 -> Data Type Conversion7/1  "<FRS_P1_04_Obj_YPos_Stdev>"
  Data Type Conversion15/1 -> Bus Creator/16
  Bus Selector/1 -> Data Type Conversion/1  "<FRS_P1_04_Msg_CheckSum>"
  Bus Selector/15 -> Data Type Conversion14/1  "<FRS_P2_04_Obj_MeasFlag>"
  Bus Selector/3 -> Data Type Conversion2/1  "<FRS_P1_04_Obj_ExstProb>"
  Bus Selector/13 -> Data Type Conversion12/1  "<FRS_P2_04_Msg_CheckSum>"
  Bus Selector/2 -> Data Type Conversion1/1  "<FRS_P1_04_Msg_AliveCounter>"
  Data Type Conversion11/1 -> Bus Creator/12
  Data Type Conversion5/1 -> Bus Creator/6
  Bus Selector/4 -> Data Type Conversion3/1  "<FRS_P1_04_Obj_XVelRel_Stdev>"
  Bus Selector/7 -> Data Type Conversion6/1  "<FRS_P1_04_Obj_MotionPattern>"
  Data Type Conversion9/1 -> Bus Creator/10
  Bus Selector/6 -> Data Type Conversion5/1  "<FRS_P1_04_Obj_ObstacleProb>"
  Data Type Conversion18/1 -> Bus Creator/19
  Bus Selector/11 -> Data Type Conversion10/1  "<FRS_P1_04_Obj_UpdateFlag>"
  Data Type Conversion17/1 -> Bus Creator/18
  Bus Selector/16 -> Data Type Conversion15/1  "<FRS_P2_04_Obj_YVelRel>"
  Data Type Conversion6/1 -> Bus Creator/7
  Bus Selector/12 -> Data Type Conversion11/1  "<FRS_P1_04_Obj_ID>"
  Data Type Conversion16/1 -> Bus Creator/17
  Bus Selector/9 -> Data Type Conversion8/1  "<FRS_P1_04_Obj_ValidFlag>"
  Bus Selector/17 -> Data Type Conversion16/1  "<FRS_P2_04_Obj_Type>"
  Bus Selector/10 -> Data Type Conversion9/1  "<FRS_P1_04_Obj_XPos_Stdev>"
  Data Type Conversion10/1 -> Bus Creator/11
  Bus Selector/14 -> Data Type Conversion13/1  "<FRS_P2_04_Msg_AliveCounter>"
  Bus Selector/19 -> Data Type Conversion18/1  "<FRS_P2_04_Obj_YPos>"
  Bus Selector/18 -> Data Type Conversion17/1  "<FRS_P2_04_Obj_XPos>"
  Bus Selector/20 -> Data Type Conversion19/1  "<FRS_P2_04_Obj_XVelRel>"
  In1/1 -> Bus Selector/1
  Bus Creator/1 -> Out1/1
  Data Type Conversion/1 -> Bus Creator/1
  Data Type Conversion2/1 -> Bus Creator/3
  Data Type Conversion13/1 -> Bus Creator/14
  Data Type Conversion1/1 -> Bus Creator/2
  Data Type Conversion4/1 -> Bus Creator/5
  Data Type Conversion3/1 -> Bus Creator/4
  Data Type Conversion7/1 -> Bus Creator/8
  Data Type Conversion8/1 -> Bus Creator/9
  Data Type Conversion14/1 -> Bus Creator/15
  Data Type Conversion19/1 -> Bus Creator/20

== system Intergration/Radar410_RX/Subsystem41/Subsystem40 ==
  In1 : Inport
  Bus Creator : BusCreator  Inputs=11  OutDataTypeStr=Bus: Radar_Status  NonVirtualBus=on
      settings: InheritFromInputs=off
  Bus Selector : BusSelector  OutputSignals=FRS_Msg_CheckSum,FRS_Msg_AliveCounter,FRS_Status_MisAlign,FRS_Status_HWErr,FRS_Status_BlkProg,FRS_Fail,FRS_MeasEnabled,FRS_Host_Yaw,FRS_HostSpeed,FRS_TimeStamp,FRS_Latency
  Data Type Conversion{,1..10} (11 alike) : DataTypeConversion  OutDataTypeStr=single
  Out1 : Outport  OutDataTypeStr=Bus: Radar_Status
  wires:
  Bus Selector/5 -> Data Type Conversion4/1  "<FRS_Status_BlkProg>"
  Bus Selector/8 -> Data Type Conversion7/1  "<FRS_Host_Yaw>"
  Bus Selector/1 -> Data Type Conversion/1  "<FRS_Msg_CheckSum>"
  Bus Selector/3 -> Data Type Conversion2/1  "<FRS_Status_MisAlign>"
  Bus Selector/2 -> Data Type Conversion1/1  "<FRS_Msg_AliveCounter>"
  Data Type Conversion5/1 -> Bus Creator/6
  Bus Selector/4 -> Data Type Conversion3/1  "<FRS_Status_HWErr>"
  Bus Selector/7 -> Data Type Conversion6/1  "<FRS_MeasEnabled>"
  Data Type Conversion9/1 -> Bus Creator/10
  Bus Selector/6 -> Data Type Conversion5/1  "<FRS_Fail>"
  Bus Selector/11 -> Data Type Conversion10/1  "<FRS_Latency>"
  Data Type Conversion6/1 -> Bus Creator/7
  Bus Selector/9 -> Data Type Conversion8/1  "<FRS_HostSpeed>"
  Bus Selector/10 -> Data Type Conversion9/1  "<FRS_TimeStamp>"
  Data Type Conversion10/1 -> Bus Creator/11
  In1/1 -> Bus Selector/1
  Bus Creator/1 -> Out1/1
  Data Type Conversion/1 -> Bus Creator/1
  Data Type Conversion2/1 -> Bus Creator/3
  Data Type Conversion1/1 -> Bus Creator/2
  Data Type Conversion4/1 -> Bus Creator/5
  Data Type Conversion3/1 -> Bus Creator/4
  Data Type Conversion7/1 -> Bus Creator/8
  Data Type Conversion8/1 -> Bus Creator/9

== system Intergration/Radar410_RX/Subsystem41/Subsystem5 ==
  In1 : Inport
  Bus Creator : BusCreator  Inputs=20  OutDataTypeStr=Bus: Obj_Data  NonVirtualBus=on
      settings: InheritFromInputs=off
  Bus Selector : BusSelector  OutputSignals=FRS_P1_05_Msg_CheckSum,FRS_P1_05_Msg_AliveCounter,FRS_P1_05_Obj_ExstProb,FRS_P1_05_Obj_XVelRel_Stdev,FRS_P1_05_Obj_XAccRel,FRS_P1_05_Obj_ObstacleProb,FRS_P1_05_Obj_MotionPattern,FRS_P1_05_Obj_YPos_Stdev,FRS_P1_05_Obj_ValidFlag,FRS_P1_05_Obj_XPos_Stdev,FRS_P1_05_Obj_UpdateFlag,FRS_P1_05_Obj_ID,FRS_P2_05_Msg_CheckSum,FRS_P2_05_Msg_AliveCounter,FRS_P2_05_Obj_MeasFlag,FRS_P2_05_Obj_YVelRel,FRS_P2_05_Obj_Type,FRS_P2_05_Obj_XPos,FRS_P2_05_Obj_YPos,FRS_P2_05_Obj_XVelRel
  Data Type Conversion{,1..19} (20 alike) : DataTypeConversion  OutDataTypeStr=single
  Out1 : Outport  OutDataTypeStr=Bus: Obj_Data
  wires:
  Data Type Conversion19/1 -> Bus Creator/20
  Data Type Conversion14/1 -> Bus Creator/15
  Data Type Conversion8/1 -> Bus Creator/9
  Data Type Conversion7/1 -> Bus Creator/8
  Data Type Conversion3/1 -> Bus Creator/4
  Data Type Conversion4/1 -> Bus Creator/5
  Data Type Conversion1/1 -> Bus Creator/2
  Data Type Conversion13/1 -> Bus Creator/14
  Data Type Conversion2/1 -> Bus Creator/3
  Data Type Conversion/1 -> Bus Creator/1
  Bus Creator/1 -> Out1/1
  In1/1 -> Bus Selector/1
  Bus Selector/20 -> Data Type Conversion19/1  "<FRS_P2_05_Obj_XVelRel>"
  Bus Selector/18 -> Data Type Conversion17/1  "<FRS_P2_05_Obj_XPos>"
  Bus Selector/19 -> Data Type Conversion18/1  "<FRS_P2_05_Obj_YPos>"
  Bus Selector/14 -> Data Type Conversion13/1  "<FRS_P2_05_Msg_AliveCounter>"
  Data Type Conversion10/1 -> Bus Creator/11
  Bus Selector/10 -> Data Type Conversion9/1  "<FRS_P1_05_Obj_XPos_Stdev>"
  Bus Selector/17 -> Data Type Conversion16/1  "<FRS_P2_05_Obj_Type>"
  Bus Selector/9 -> Data Type Conversion8/1  "<FRS_P1_05_Obj_ValidFlag>"
  Data Type Conversion16/1 -> Bus Creator/17
  Bus Selector/12 -> Data Type Conversion11/1  "<FRS_P1_05_Obj_ID>"
  Data Type Conversion6/1 -> Bus Creator/7
  Bus Selector/16 -> Data Type Conversion15/1  "<FRS_P2_05_Obj_YVelRel>"
  Data Type Conversion17/1 -> Bus Creator/18
  Bus Selector/11 -> Data Type Conversion10/1  "<FRS_P1_05_Obj_UpdateFlag>"
  Data Type Conversion18/1 -> Bus Creator/19
  Bus Selector/6 -> Data Type Conversion5/1  "<FRS_P1_05_Obj_ObstacleProb>"
  Data Type Conversion9/1 -> Bus Creator/10
  Bus Selector/7 -> Data Type Conversion6/1  "<FRS_P1_05_Obj_MotionPattern>"
  Bus Selector/4 -> Data Type Conversion3/1  "<FRS_P1_05_Obj_XVelRel_Stdev>"
  Data Type Conversion5/1 -> Bus Creator/6
  Data Type Conversion11/1 -> Bus Creator/12
  Bus Selector/2 -> Data Type Conversion1/1  "<FRS_P1_05_Msg_AliveCounter>"
  Bus Selector/13 -> Data Type Conversion12/1  "<FRS_P2_05_Msg_CheckSum>"
  Bus Selector/3 -> Data Type Conversion2/1  "<FRS_P1_05_Obj_ExstProb>"
  Bus Selector/15 -> Data Type Conversion14/1  "<FRS_P2_05_Obj_MeasFlag>"
  Bus Selector/1 -> Data Type Conversion/1  "<FRS_P1_05_Msg_CheckSum>"
  Data Type Conversion15/1 -> Bus Creator/16
  Bus Selector/8 -> Data Type Conversion7/1  "<FRS_P1_05_Obj_YPos_Stdev>"
  Bus Selector/5 -> Data Type Conversion4/1  "<FRS_P1_05_Obj_XAccRel>"
  Data Type Conversion12/1 -> Bus Creator/13
